simulink model "Exercitiul4_3"  (R2016a)
settings: Solver=VariableStepDiscrete  StartTime=0.0  StopTime=1000  RelTol=1e-3
undefined symbols (not defined in the file): m, n
settings Model: Creator=Cristina  LastModifiedBy=Cristina

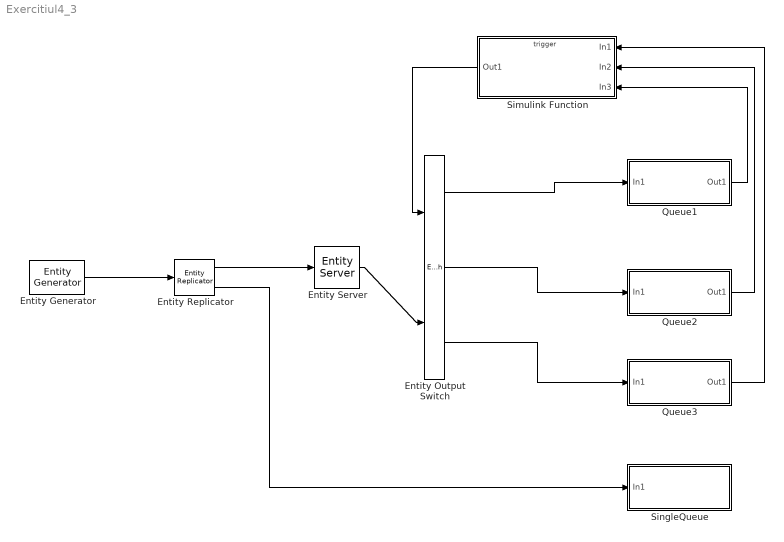
== system Exercitiul4_3 ==
  Entity Output Switch : EntityOutputSwitch  InputPortMessageModes=m,m  OutputPortMessageModes=m,m,m  NumberOutputPorts=3  SwitchingCriterion=From control port  SwitchAttributeName=Attribute1
      settings: InputPortMap=u0,u1  OutputPortMap=o0,o1,o2
  Entity Generator : EntityGenerator  OutputPortMessageModes=m  IntergenerationTimeAction=|  GenerateAction=|  AttributeName=ServiceTime  EntityType=Structured  EntityTypeName=Entity
      IntergenerationTimeAction=|
      | persistent init
      | if (isempty(init))
      |     rng(177);
      |     init = true;
      | end
      | 
      | pr = rand;
      | if(pr <=0.29)
      |     entity.ServiceTime = exprnd(1);
      | else if (pr <=0.56)
      |             entity.ServiceTime = exprnd(2);
      |      else
      |         entity.ServiceTime = exprnd(5);
      | end
      GenerateAction=|
      | persistent init
      | if (isempty(init))
      |     rng(177);
      |     init = true;
      | end
      | 
      | pr = rand;
      | if(pr <=0.29)
      |     entity.ServiceTime = exprnd(1);
      | else if (pr <=0.56)
      |             entity.ServiceTime = exprnd(2);
      |      else
      |         entity.ServiceTime = exprnd(5);
      | end
  Entity Replicator : EntityReplicator  InputPortMessageModes=m  OutputPortMessageModes=m,m
  Entity Server : EntityServer  InputPortMessageModes=m  OutputPortMessageModes=m  Capacity=3
  Queue1 : Subsystem
  Queue2 : Subsystem
  Queue3 : Subsystem
  Simulink Function : Subsystem  TreatAsAtomicUnit=on
  SingleQueue : Subsystem
  wires:
  Entity Generator/1 -> Entity Replicator/1
  Entity Replicator/1 -> Entity Server/1
  Entity Server/1 -> Entity Output Switch/2
  Entity Replicator/2 -> SingleQueue/1(In1)
  Queue1/1(Out1) -> Simulink Function/3(In3)
  Queue2/1(Out1) -> Simulink Function/2(In2)
  Queue3/1(Out1) -> Simulink Function/1(In1)
  Simulink Function/1(Out1) -> Entity Output Switch/1
  Entity Output Switch/1 -> Queue1/1(In1)
  Entity Output Switch/2 -> Queue2/1(In1)
  Entity Output Switch/3 -> Queue3/1(In1)

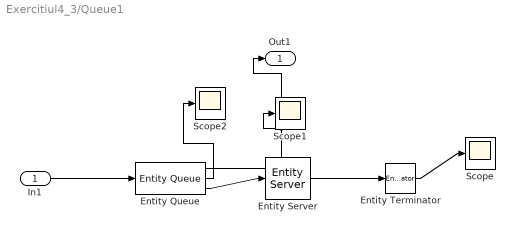
== system Exercitiul4_3/Queue1 ==
  In1 : Inport
  Entity Queue : EntityQueue  InputPortMessageModes=m  OutputPortMessageModes=n,n,m  NumberEntitiesInBlock=on  AverageWait=on
      settings: OutputPortMap=o1,o2,o5
  Entity Server : EntityServer  InputPortMessageModes=m  OutputPortMessageModes=m  Capacity=1
  Entity Terminator : EntityTerminator  InputPortMessageModes=m  NumberEntitiesArrived=on
      settings: OutputPortMap=o0
  Scope : Scope
  Scope1 : Scope
  Scope2 : Scope
  Out1 : Outport
  wires:
  In1/1 -> Entity Queue/1
  Entity Queue/3 -> Entity Server/1
  Entity Server/1 -> Entity Terminator/1
  Entity Terminator/1 -> Scope/1
  Entity Queue/1 -> Out1/1, Scope1/1
  Entity Queue/2 -> Scope2/1

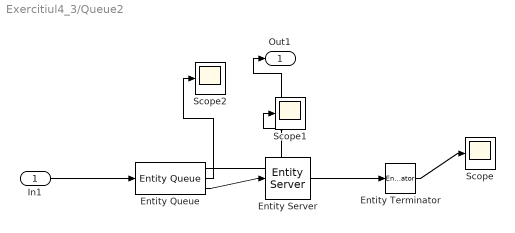
== system Exercitiul4_3/Queue2 ==
  In1 : Inport
  Entity Queue : EntityQueue  InputPortMessageModes=m  OutputPortMessageModes=n,n,m  NumberEntitiesInBlock=on  AverageWait=on
      settings: OutputPortMap=o1,o2,o5
  Entity Server : EntityServer  InputPortMessageModes=m  OutputPortMessageModes=m  Capacity=1
  Entity Terminator : EntityTerminator  InputPortMessageModes=m  NumberEntitiesArrived=on
      settings: OutputPortMap=o0
  Scope : Scope
  Scope1 : Scope
  Scope2 : Scope
  Out1 : Outport
  wires:
  In1/1 -> Entity Queue/1
  Entity Queue/3 -> Entity Server/1
  Entity Server/1 -> Entity Terminator/1
  Entity Terminator/1 -> Scope/1
  Entity Queue/1 -> Out1/1, Scope1/1
  Entity Queue/2 -> Scope2/1

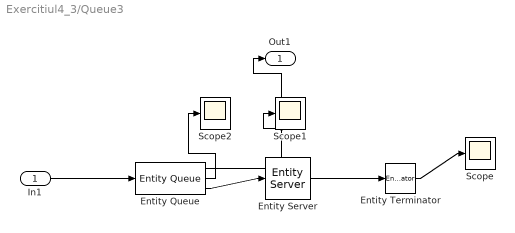
== system Exercitiul4_3/Queue3 ==
  In1 : Inport
  Entity Queue : EntityQueue  InputPortMessageModes=m  OutputPortMessageModes=n,n,m  NumberEntitiesInBlock=on  AverageWait=on
      settings: OutputPortMap=o1,o2,o5
  Entity Server : EntityServer  InputPortMessageModes=m  OutputPortMessageModes=m  Capacity=1
  Entity Terminator : EntityTerminator  InputPortMessageModes=m  NumberEntitiesArrived=on
      settings: OutputPortMap=o0
  Scope : Scope
  Scope1 : Scope
  Scope2 : Scope
  Out1 : Outport
  wires:
  In1/1 -> Entity Queue/1
  Entity Queue/3 -> Entity Server/1
  Entity Server/1 -> Entity Terminator/1
  Entity Terminator/1 -> Scope/1
  Entity Queue/1 -> Out1/1, Scope1/1
  Entity Queue/2 -> Scope2/1

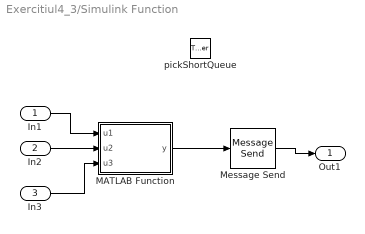
== system Exercitiul4_3/Simulink Function ==
  In1 : Inport
  In2 : Inport  Port=2
  In3 : Inport  Port=3
  pickShortQueue : TriggerPort  TriggerType=function-call  IsSimulinkFunction=on  FunctionName=pickShortQueue  VariantControl=Variant
  MATLAB Function : MATLAB Function  TreatAsAtomicUnit=on
  Message Send : MessageSend  OutputPortMessageModes=m
      settings: InputPortMap=u1
  Out1 : Outport
  wires:
  Message Send/1 -> Out1/1
  In1/1 -> MATLAB Function/1(u1)
  In2/1 -> MATLAB Function/2(u2)
  In3/1 -> MATLAB Function/3(u3)
  MATLAB Function/1(y) -> Message Send/1

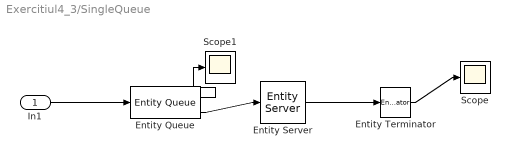
== system Exercitiul4_3/SingleQueue ==
  In1 : Inport
  Entity Queue : EntityQueue  InputPortMessageModes=m  OutputPortMessageModes=n,m  AverageWait=on
      settings: OutputPortMap=o2,o5
  Entity Server : EntityServer  InputPortMessageModes=m  OutputPortMessageModes=m  Capacity=3
  Entity Terminator : EntityTerminator  InputPortMessageModes=m  NumberEntitiesArrived=on
      settings: OutputPortMap=o0
  Scope : Scope
  Scope1 : Scope
  wires:
  Entity Queue/2 -> Entity Server/1
  Entity Server/1 -> Entity Terminator/1
  Entity Terminator/1 -> Scope/1
  In1/1 -> Entity Queue/1
  Entity Queue/1 -> Scope1/1

== matlab function Exercitiul4_3/Simulink Function/MATLAB Function ==
  data: u1 input; y output; u2 input; u3 input
function y = fct(u1,u2,u3)
%#codegen

[a,y] = min([u3,u2,u1]);
